simulink model "ultrasonic_task"  (Simulink 3.00)
libraries: mathlib x4, arclib x1

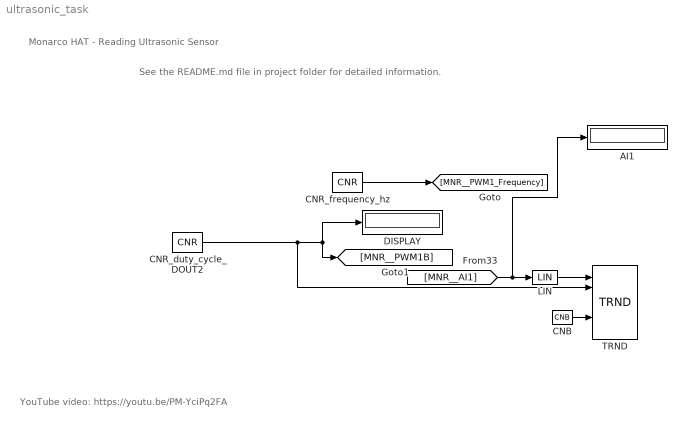
== system ultrasonic_task ==
  note: See the README.md file in project folder for detailed information.
  note: Monarco HAT - Reading Ultrasonic Sensor
  note: YouTube video: https://youtu.be/PM-YciPq2FA
  AI1 : Display
      settings: Format=short  Suffix=V
  CNB : mathlib/CNB  YCN=on
  CNR_duty_cycle_DOUT2 : mathlib/CNR  ycn=0.4
  CNR_frequency_hz : mathlib/CNR  ycn=40000
  DISPLAY : Display
      settings: Format=short  Suffix=V
  LIN : mathlib/LIN  u1=0  y1=3  u2=10  y2=29
  TRND : arclib/TRND  n=1  l=5000  btype=8: Double  ptype1=1: Store  ptype2=1: Store  ptype3=1: Store  ptype4=1: Store  pfac=50  afac=0  arc=0  id=1  Title=Trend Title  timesrc=1
  wires:
  CNB/1 -> TRND/5
  CNR_duty_cycle_DOUT2/1 -> DISPLAY/1, [MNR__PWM1B], TRND/2
  CNR_frequency_hz/1 -> [MNR__PWM1_Frequency]
  [MNR__AI1] -> AI1/1, LIN/1
  LIN/1 -> TRND/1
